simulink model "get_x0u0unc"  (Simulink 3.00)
settings: Solver=ode4  StartTime=0.0  StopTime=10.0  FixedStep=0.02  RelTol=1e-3
undefined symbols (not defined in the file or in its folder): Alt, dalt_err, dMach_err, Mach
settings Model: SaveState=on  LastModifiedBy=hkg

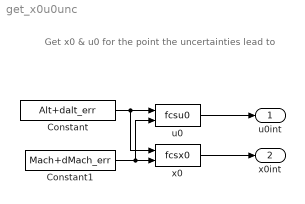
== system get_x0u0unc ==
  note: Get x0 & u0 for the point the
      | uncertainties lead to
  Constant : Constant  Value=Alt+dalt_err
  Constant1 : Constant  Value=Mach+dMach_err
  u0 : S-Function  FunctionName=fcsu0  PortCounts=[]  SFunctionModules=''
  x0 : S-Function  FunctionName=fcsx0  PortCounts=[]  SFunctionModules=''
  u0int : Outport  Port=1
  x0int : Outport  Port=2
  wires:
  x0/1 -> x0int/1
  Constant/1 -> u0/1, x0/1
  Constant1/1 -> x0/2, u0/2
  u0/1 -> u0int/1
